simulink model "testbench_or_gyro_control"  (R2016a)
settings: Solver=FixedStepAuto  StartTime=0.0  StopTime=10.0  RelTol=1e-3
libraries: legoev3lib x2
settings Model: SimulationMode=external  ExtModeTrigDuration=2  Creator=Shobhit  LastModifiedBy=Shobhit
settings SolverCC: PositivePriorityOrder=on
settings OptimizationCC: OptimizeModelRefInitCode=on  LifeSpan=1  MaxStackSize=64
settings HardwareCC: ProdBitPerPointer=32  ProdLargestAtomicInteger=Long  ProdWordSize=32  ProdHWDeviceType=ARM Compatible->ARM 9  UseEmbeddedCoderFeatures=off  UseSimulinkCoderFeatures=off
settings RTWCC: SystemTargetFile=ert.tlc  HardwareBoard=LEGO MINDSTORMS EV3  TemplateMakefile=ert_default_tmf  GenerateReport=on  Toolchain=Sourcery G++ Lite v2009q3  IncludeHyperlinkInReport=on  LaunchReport=on  GenerateTraceInfo=on  GenerateTraceReport=on  GenerateTraceReportSl=on  GenerateTraceReportSf=on  GenerateTraceReportEml=on
settings CodeAppCC: ForceParamTrailComments=on  IgnoreCustomStorageClasses=off  OperatorAnnotations=on  SimulinkDataObjDesc=on  SFDataObjDesc=on  MATLABFcnDesc=on  InsertBlockDesc=on  MATLABSourceComments=on
settings ERTTargetCC: SupportContinuousTime=on  SupportNonInlinedSFcns=on  SupportVariableSizeSignals=on

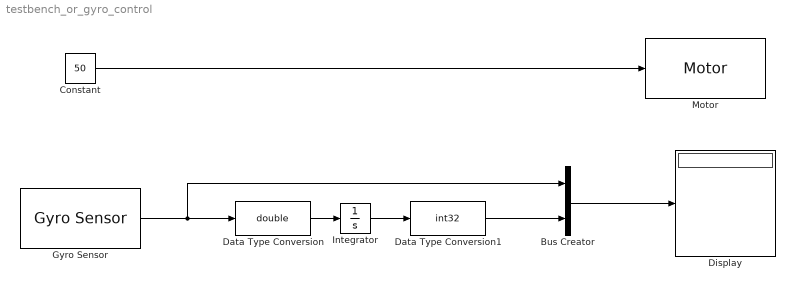
== system testbench_or_gyro_control ==
  Bus Creator : BusCreator  Inputs=2
  Constant : Constant  Value=50
  Data Type Conversion : DataTypeConversion  OutDataTypeStr=double  RndMeth=Ceiling
  Data Type Conversion1 : DataTypeConversion  OutDataTypeStr=int32  RndMeth=Ceiling
  Display : Display
  Gyro Sensor : legoev3lib/Gyro Sensor  portNumber=1  sampleTime=0.1
  Integrator : Integrator
  Motor : legoev3lib/Motor  sportNumber=A  sstopAction=Brake
  wires:
  Constant/1 -> Motor/1
  Gyro Sensor/1 -> Data Type Conversion/1, Bus Creator/1
  Integrator/1 -> Data Type Conversion1/1
  Bus Creator/1 -> Display/1
  Data Type Conversion/1 -> Integrator/1
  Data Type Conversion1/1 -> Bus Creator/2
